simulink model "AMbaoluo"  (R2017b)
settings: Solver=VariableStepAuto  StartTime=0.0  StopTime=10.0  MaxStep=1e-4  RelTol=1e-3
libraries: dsparch4 x2
settings Model: Creator=DELL  LastModifiedBy=DELL

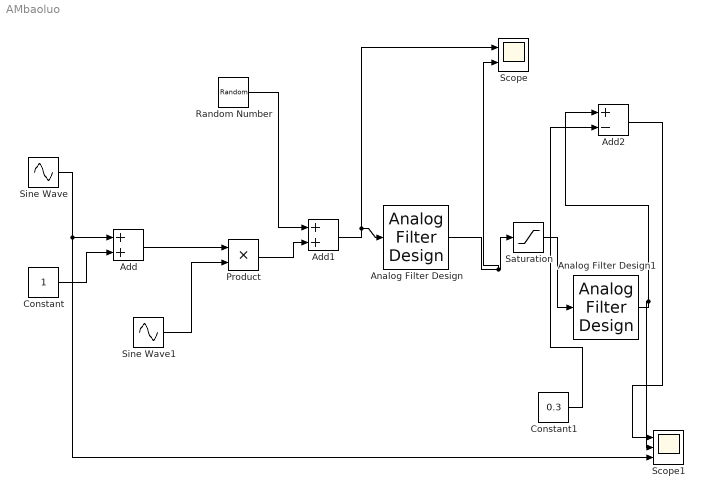
== system AMbaoluo ==
  Add : Sum
  Add1 : Sum
  Add2 : Sum  Inputs=+-
  Analog Filter Design : dsparch4/Analog Filter Design  method=Butterworth  filttype=Bandpass  N=8  Wlo=90  Whi=110  Rp=2  Rs=40
  Analog Filter Design1 : dsparch4/Analog Filter Design  method=Butterworth  filttype=Lowpass  N=8  Wlo=10  Whi=250  Rp=2  Rs=40
  Constant : Constant
  Constant1 : Constant  Value=0.3
  Product : Product
  Random Number : RandomNumber  SampleTime=0.01
  Saturation : Saturate  UpperLimit=inf  LowerLimit=0
  Scope : Scope  NumInputPorts=2
  Scope1 : Scope  NumInputPorts=3
  Sine Wave : Sin  Frequency=10  SampleTime=0
  Sine Wave1 : Sin  Frequency=100  SampleTime=0
  wires:
  Constant/1 -> Add/2
  Sine Wave1/1 -> Product/2
  Add/1 -> Product/1
  Random Number/1 -> Add1/1
  Saturation/1 -> Analog Filter Design1/1
  Analog Filter Design1/1 -> Scope1/2, Add2/1
  Constant1/1 -> Add2/2
  Product/1 -> Add1/2
  Analog Filter Design/1 -> Scope/2, Saturation/1
  Add2/1 -> Scope1/1
  Sine Wave/1 -> Add/1, Scope1/3
  Add1/1 -> Analog Filter Design/1, Scope/1
